simulink model "plantaMalhaInterna"  (R2018b)
settings: Solver=VariableStepAuto  StartTime=0.0  StopTime=10.0  RelTol=1e-3
values from neighbouring files (symbols this model uses):
  den = [1 - 2.981694681338594 2.963566104560976 -0.981871423222382]    [Main_Malha_Externa.m]    (also in Main_Malha_Externa_referencia.m; main.m = -0.995; main_malha_interna.m = -0.995; otimiza_Dir.m = -0.9975)
  num = [1.104392655054829e-08 3.313177965164485e-08 3.313177965164485e-08 1.104392655054829e-08]    [Main_Malha_Externa.m]    (also in Main_Malha_Externa_referencia.m; main.m = 2.868e-05; main_malha_interna.m = 2.868e-05; otimiza_Dir.m = 2.514e-05)
  x = fmincon(@otimiza_PIDF,x,[],[],[],[],[0 0 0 0],[inf inf inf inf],@QQQ,options)    [Main_Malha_Externa.m]    (also in Main_Malha_Externa_referencia.m = fmincon(@otimiza_PIDF_referencia,x,[],[],[],[],[0 0 0 0],[in; main.m = fmincon(@otimiza_Esq,x,[],[],[],[],[0 0 0],[inf inf 1400],@Q; main_malha_interna.m = fmincon(@otimiza_Esq,x,[],[],[],[],[0 0 0],[inf inf 1400],@Q; otimiza_Dir.m = X)
settings Model: Creator=vitor  LastModifiedBy=vitor

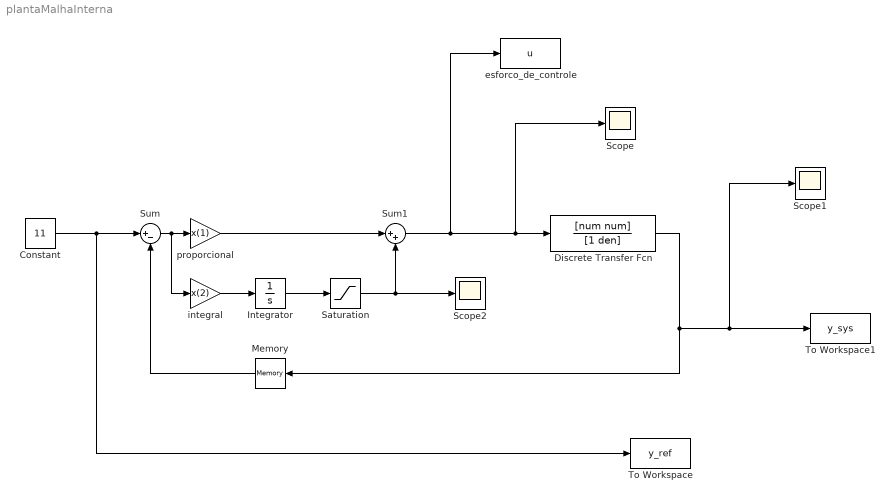
== system plantaMalhaInterna ==
  Constant : Constant  Value=11
  Discrete Transfer Fcn : DiscreteTransferFcn  Numerator=[num num]  Denominator=[1 den]  SampleTime=0.001
  Integrator : Integrator
  Memory : Memory
  Saturation : Saturate  UpperLimit=x(3)  LowerLimit=0
  Scope : Scope
  Scope1 : Scope
  Scope2 : Scope
  Sum : Sum  Inputs=|+-
  Sum1 : Sum  Inputs=|++
  To Workspace : ToWorkspace  VariableName=y_ref  SampleTime=-1
  To Workspace1 : ToWorkspace  VariableName=y_sys  SampleTime=-1
  esforco_de_controle : ToWorkspace  VariableName=u  SampleTime=-1
  integral : Gain  Gain=x(2)
  proporcional : Gain  Gain=x(1)
  wires:
  Integrator/1 -> Saturation/1
  Sum/1 -> integral/1, proporcional/1
  integral/1 -> Integrator/1
  Discrete Transfer Fcn/1 -> Memory/1, To Workspace1/1, Scope1/1
  Saturation/1 -> Scope2/1, Sum1/2
  Memory/1 -> Sum/2
  Sum1/1 -> esforco_de_controle/1, Scope/1, Discrete Transfer Fcn/1
  Constant/1 -> To Workspace/1, Sum/1
  proporcional/1 -> Sum1/1
